simulink model "graph2"  (R2021b)
settings: Solver=VariableStepAuto  StartTime=0.0  StopTime=10.0  RelTol=1e-3
settings Model: Creator=hamza  LastModifiedBy=hamza

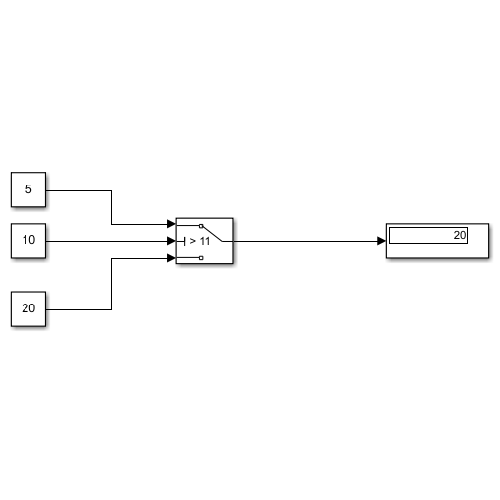
[thumbnail: Simulink's stored preview of the top-level diagram]
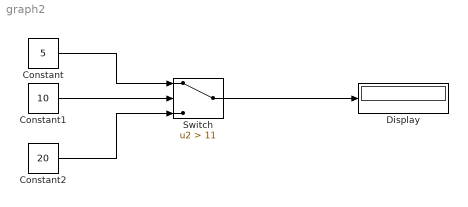
== system graph2 ==
  Constant : Constant  Value=5
  Constant1 : Constant  Value=10
  Constant2 : Constant  Value=20
  Display : Display
  Switch : Switch  Criteria=u2 > Threshold  Threshold=11
  wires:
  Constant/1 -> Switch/1
  Constant1/1 -> Switch/2
  Constant2/1 -> Switch/3
  Switch/1 -> Display/1
